simulink model "test_libMdl_BiasEstimator"  (R2019b)
settings: Solver=FixedStepAuto  StartTime=0.0  StopTime=50  FixedStep=0.002  RelTol=1e-3
libraries: libMdl_InsBiasEstimator x1
settings Model: Creator=Hanno  LastModifiedBy=Hanno
settings DataIOCC: SaveOutput=off  SignalLogging=off  DSMLogging=off  SaveTime=off  ReturnWorkspaceOutputs=off

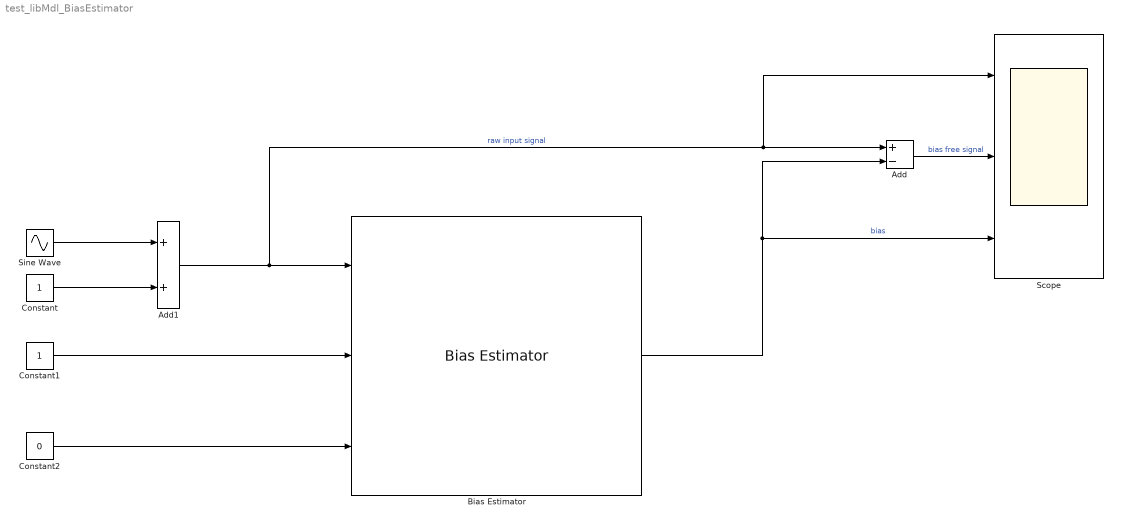
== system test_libMdl_BiasEstimator ==
  Add : Sum  Inputs=+-
  Add1 : Sum
  Bias Estimator : libMdl_InsBiasEstimator/Bias Estimator  mv_bias_gain=0.001
  Constant : Constant
  Constant1 : Constant
  Constant2 : Constant  Value=0
  Scope : Scope  NumInputPorts=3
  Sine Wave : Sin  Frequency=20  SampleTime=0
  wires:
  Sine Wave/1 -> Add1/1
  Constant/1 -> Add1/2
  Constant1/1 -> Bias Estimator/2
  Constant2/1 -> Bias Estimator/3
  Bias Estimator/1 -> Add/2, Scope/3  "bias"
  Add/1 -> Scope/2  "bias free signal"
  Add1/1 -> Bias Estimator/1, Scope/1, Add/1  "raw input signal"
